simulink library "lowFreqFlowData_ul"  (R2018b)
settings: Solver=VariableStepAuto  StartTime=0.0  StopTime=10.0  RelTol=1e-3
undefined symbols (not defined in the file): flw
settings Model: Creator=M.Cobb  LastModifiedBy=mcobb

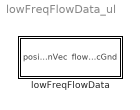
== system lowFreqFlowData_ul ==
  lowFreqFlowData : Subsystem  VariantControl=VSS_flowCalculation_constXYZT  mask{flw=flw}
      mask prompts: flw "Low Freq Flow obj (eg ENV.CNAPS)"

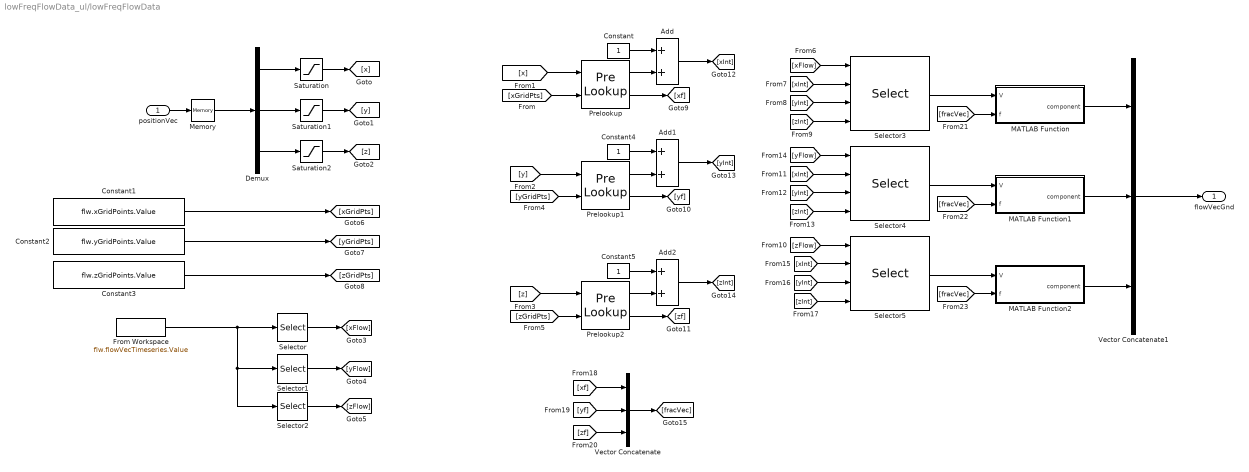
== system lowFreqFlowData_ul/lowFreqFlowData ==
  positionVec : Inport  PortDimensions=[3 1]
  Add : Sum
  Add1 : Sum
  Add2 : Sum
  Constant : Constant
  Constant1 : Constant  Value=flw.xGridPoints.Value
  Constant2 : Constant  Value=flw.yGridPoints.Value
  Constant3 : Constant  Value=flw.zGridPoints.Value
  Constant4 : Constant
  Constant5 : Constant
  Demux : Demux  Outputs=3
  From Workspace : FromWorkspace  VariableName=flw.flowVecTimeseries.Value  SampleTime=0
  MATLAB Function : MATLAB Function  TreatAsAtomicUnit=on
  MATLAB Function1 : MATLAB Function  TreatAsAtomicUnit=on
  MATLAB Function2 : MATLAB Function  TreatAsAtomicUnit=on
  Memory : Memory  InitialCondition=[0 0 0]'
  Prelookup : PreLookup  BreakpointsDataSource=Input port  BreakpointsData=[10:10:110]  BeginIndexSearchUsingPreviousIndexResult=on  ExtrapMethod=Linear
      settings: InputPortMap=u0,p1
  Prelookup1 : PreLookup  BreakpointsDataSource=Input port  BreakpointsData=[10:10:110]  BeginIndexSearchUsingPreviousIndexResult=on  ExtrapMethod=Linear
      settings: InputPortMap=u0,p1
  Prelookup2 : PreLookup  BreakpointsDataSource=Input port  BreakpointsData=[10:10:110]  BeginIndexSearchUsingPreviousIndexResult=on  ExtrapMethod=Linear
      settings: InputPortMap=u0,p1
  Saturation : Saturate  UpperLimit=max(flw.xGridPoints.Value)  LowerLimit=min(flw.xGridPoints.Value)
  Saturation1 : Saturate  UpperLimit=max(flw.yGridPoints.Value)  LowerLimit=min(flw.yGridPoints.Value)
  Saturation2 : Saturate  UpperLimit=max(flw.zGridPoints.Value)  LowerLimit=min(flw.zGridPoints.Value)
  Selector : Selector  NumberOfDimensions=4  InputPortWidth=3  IndexOptions=Select all,Select all,Select all,Index vector (dialog)  Indices=[1 3],1,1,1  OutputSizes=1,1,1,1
  Selector1 : Selector  NumberOfDimensions=4  InputPortWidth=3  IndexOptions=Select all,Select all,Select all,Index vector (dialog)  Indices=[1 3],1,1,2  OutputSizes=1,1,1,1
  Selector2 : Selector  NumberOfDimensions=4  InputPortWidth=3  IndexOptions=Select all,Select all,Select all,Index vector (dialog)  Indices=[1 3],1,1,3  OutputSizes=1,1,1,1
  Selector3 : Selector  NumberOfDimensions=3  InputPortWidth=3  IndexOptions=Starting index (port),Starting index (port),Starting index (port)  Indices=[1 3],1,1  OutputSizes=2,2,2
  Selector4 : Selector  NumberOfDimensions=3  InputPortWidth=3  IndexOptions=Starting index (port),Starting index (port),Starting index (port)  Indices=[1 3],1,1  OutputSizes=2,2,2
  Selector5 : Selector  NumberOfDimensions=3  InputPortWidth=3  IndexOptions=Starting index (port),Starting index (port),Starting index (port)  Indices=[1 3],1,1  OutputSizes=2,2,2
  Vector Concatenate : Concatenate  NumInputs=3
  Vector Concatenate1 : Concatenate  NumInputs=3
  flowVecGnd : Outport
  wires:
  Add2/1 -> [zInt]
  Constant5/1 -> Add2/1
  Add1/1 -> [yInt]
  Constant4/1 -> Add1/1
  Add/1 -> [xInt]
  Constant/1 -> Add/1
  positionVec/1 -> Memory/1
  Demux/1 -> Saturation/1
  Demux/2 -> Saturation1/1
  Demux/3 -> Saturation2/1
  Saturation/1 -> [x]
  Saturation1/1 -> [y]
  Saturation2/1 -> [z]
  From Workspace/1 -> Selector2/1, Selector1/1, Selector/1
  Selector/1 -> [xFlow]
  Selector1/1 -> [yFlow]
  Selector2/1 -> [zFlow]
  Constant1/1 -> [xGridPts]
  Constant2/1 -> [yGridPts]
  Constant3/1 -> [zGridPts]
  [xGridPts] -> Prelookup/2
  [x] -> Prelookup/1
  [y] -> Prelookup1/1
  [z] -> Prelookup2/1
  [yGridPts] -> Prelookup1/2
  [zGridPts] -> Prelookup2/2
  Prelookup/2 -> [xf]
  Prelookup1/2 -> [yf]
  Prelookup2/2 -> [zf]
  [xFlow] -> Selector3/1
  Prelookup/1 -> Add/2
  Prelookup1/1 -> Add1/2
  Prelookup2/1 -> Add2/2
  [xInt] -> Selector3/2
  [yInt] -> Selector3/3
  [zInt] -> Selector3/4
  [zInt] -> Selector4/4
  [yInt] -> Selector4/3
  [xInt] -> Selector4/2
  [yFlow] -> Selector4/1
  [zFlow] -> Selector5/1
  [xInt] -> Selector5/2
  [yInt] -> Selector5/3
  [zInt] -> Selector5/4
  [yf] -> Vector Concatenate/2
  [xf] -> Vector Concatenate/1
  [zf] -> Vector Concatenate/3
  Vector Concatenate/1 -> [fracVec]
  Selector3/1 -> MATLAB Function/1(V)
  [fracVec] -> MATLAB Function/2(f)
  [fracVec] -> MATLAB Function1/2(f)
  Selector4/1 -> MATLAB Function1/1(V)
  [fracVec] -> MATLAB Function2/2(f)
  Selector5/1 -> MATLAB Function2/1(V)
  MATLAB Function1/1(component) -> Vector Concatenate1/2
  MATLAB Function2/1(component) -> Vector Concatenate1/3
  MATLAB Function/1(component) -> Vector Concatenate1/1
  Vector Concatenate1/1 -> flowVecGnd/1
  Memory/1 -> Demux/1

== matlab function lowFreqFlowData_ul/lowFreqFlowData/MATLAB Function1 ==
  data: V input; component output; f input
function  component= fcn(V,f)

component = ...
    (1-f(1))*(1-f(2))*(1-f(3))*V(1,1,1)+...
    (1-f(1))*(1-f(2))*(  f(3))*V(1,1,2)+...
    (1-f(1))*(  f(2))*(1-f(3))*V(1,2,1)+...
    (  f(1))*(1-f(2))*(1-f(3))*V(2,1,1)+...
    (1-f(1))*(  f(2))*(  f(3))*V(1,2,2)+...
    (  f(1))*(1-f(2))*(  f(3))*V(2,1,2)+...
    (  f(1))*(  f(2))*(1-f(3))*V(2,2,1)+...
    (  f(1))*(  f(2))*(  f(3))*V(2,2,2);

== matlab function lowFreqFlowData_ul/lowFreqFlowData/MATLAB Function ==
  data: V input; component output; f input
function  component= fcn(V,f)

component = ...
    (1-f(1))*(1-f(2))*(1-f(3))*V(1,1,1)+...
    (1-f(1))*(1-f(2))*(  f(3))*V(1,1,2)+...
    (1-f(1))*(  f(2))*(1-f(3))*V(1,2,1)+...
    (  f(1))*(1-f(2))*(1-f(3))*V(2,1,1)+...
    (1-f(1))*(  f(2))*(  f(3))*V(1,2,2)+...
    (  f(1))*(1-f(2))*(  f(3))*V(2,1,2)+...
    (  f(1))*(  f(2))*(1-f(3))*V(2,2,1)+...
    (  f(1))*(  f(2))*(  f(3))*V(2,2,2);

== matlab function lowFreqFlowData_ul/lowFreqFlowData/MATLAB Function2 ==
  data: V input; component output; f input
function  component= fcn(V,f)

component = ...
    (1-f(1))*(1-f(2))*(1-f(3))*V(1,1,1)+...
    (1-f(1))*(1-f(2))*(  f(3))*V(1,1,2)+...
    (1-f(1))*(  f(2))*(1-f(3))*V(1,2,1)+...
    (  f(1))*(1-f(2))*(1-f(3))*V(2,1,1)+...
    (1-f(1))*(  f(2))*(  f(3))*V(1,2,2)+...
    (  f(1))*(1-f(2))*(  f(3))*V(2,1,2)+...
    (  f(1))*(  f(2))*(1-f(3))*V(2,2,1)+...
    (  f(1))*(  f(2))*(  f(3))*V(2,2,2);
